simulink model "DescreteModel"  (R2020b)
settings: Solver=FixedStepAuto  StartTime=0.0  StopTime=5  FixedStep=0.0001  RelTol=1e-3
InitFcn:
  | run("NonLinearModelParameters")
  | 
  | run('model_disc_controller_creator.m')
values from neighbouring files (symbols this model uses):
  B = 3.4    [NonLinearModelParameters.m]
  K_tau = 42e-3    (= 0.042)    [NonLinearModelParameters.m]
  n_1 = 1/3    (= 0.333333333333)    [NonLinearModelParameters.m]
  r_3 = 0.01571    [NonLinearModelParameters.m]
undefined symbols (not defined in the file or in its folder): cont_den, cont_num, CoulombAndViscousFriction, CurrentOffset, Delta, discrete_constants, J_eq, SignOfVelocity, T_sample
libraries: simulink x1
settings Model: Creator=jonas  LastModifiedBy=Bens PC

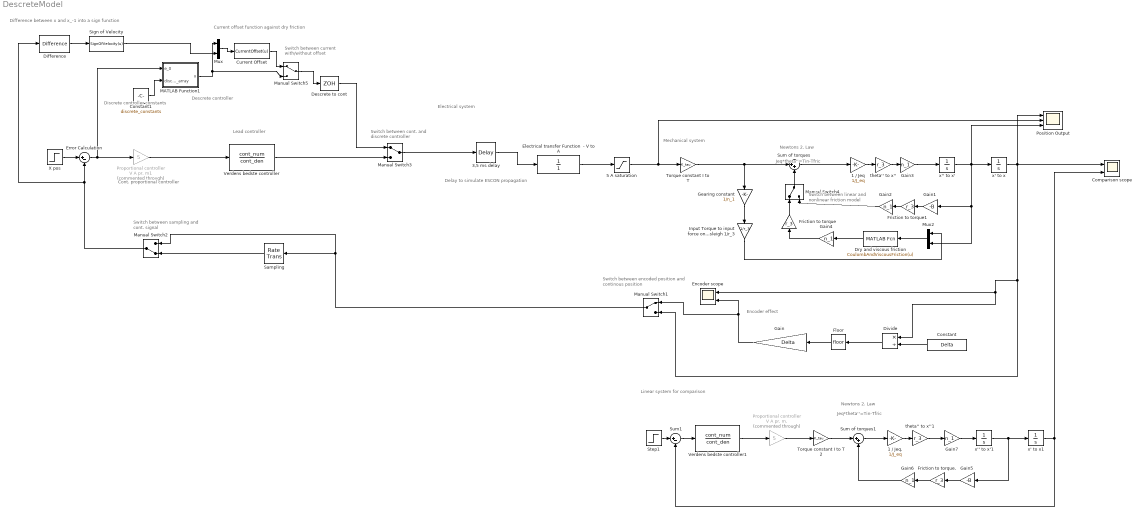
== system DescreteModel ==
  note: Discrete controller constants
  note: Difference between x and x_-1 into a sign function
  note: Linear system for comparison
  note: Switch between linear
      | and nonlinear friction model
  note: Delay to simulate ESCON propagation
  note: Switch between
      | current with/without offset
  note: Switch between sampling
      | and cont. signal
  note: Electrical system
  note: Switch between cont.
      | and discrete controller
  note: Current offset function against dry friction
  note: Cont. proportional
      | controller
  note: Switch between encoded position and
      | continous position
  note: Newtons 2. Law
  note: Mechanical system
  note: Encoder effect
  note: Jeq*theta''=Tin-Tfric
  note: Descrete controller
  note: Newtons 2. Law
  note: Jeq*theta''=Tin-Tfric
  note: Lead
      | controller
  1 / Jeq : Gain  Gain=1/J_eq
  1 / Jeq. : Gain  Gain=1/J_eq
  3,5 ms delay : TransportDelay  DelayTime=0.0035
  5 A saturation : Saturate  UpperLimit=5  LowerLimit=-5
  Comparison scope : Scope  NumInputPorts=2
  Constant : Constant  Value=Delta
  Constant1 : Constant  Value=discrete_constants
  Current Offset : MATLABFcn  MATLABFcn=CurrentOffset(u)  OutputDimensions=1
  Descrete to cont : ZeroOrderHold  SampleTime=T_sample
  Difference : simulink/Discrete/Difference  ICPrevInput=0.0  OutMin=[]  OutMax=[]  OutDataType=fixdt(1, 16)  OutScaling=2^-10  DoSatur=off
  Divide : Product  Inputs=*/
  Dry and viscous friction : MATLABFcn  MATLABFcn=CoulombAndViscousFriction(u)  OutputDimensions=1
  Electrical transfer Function  - V to A : TransferFcn  Denominator=[1]
  Encoder scope : Scope  NumInputPorts=2
  Error Calculation : Sum  Inputs=|+-
  Floor : Rounding
  Friction to torque : Gain  Gain=r_3
  Friction to torque. : Gain  Gain=r_3
  Friction to torque1 : Gain  Gain=r_3
  Gain : Gain  Gain=Delta
  Gain1 : Gain  Gain=-B
  Gain{2..4,6..7} (5 alike) : Gain  Gain=n_1
  Gain5 : Gain  Gain=-B
  Gearing constant : Gain  Gain=1/n_1
  Input Torque to input force on sleigh 1/r_3 : Gain  Gain=1/r_3
  MATLAB Function1 : MATLAB Function  TreatAsAtomicUnit=on
  Manual Switch{1,3..5} (4 alike) : ManualSwitch
  Manual Switch2 : ManualSwitch  CurrentSetting=0
  Mux : Mux  Inputs=2
  Mux2 : Mux  Inputs=2
  Position Output : Scope  NumInputPorts=3
  Proportional controller V A pr. m. : Gain  Commented=through  Gain=5
  Proportional controller V A pr. m1 : Gain  Commented=through  Gain=5
  "Sampling " : RateTransition  OutPortSampleTime=T_sample
  Sign of Velocity : MATLABFcn  MATLABFcn=SignOfVelocity(u)  OutputDimensions=1
  Step1 : Step  Time=0  After=0.5  SampleTime=0
  Sum of torques : Sum  Inputs=|++
  Sum of torques1 : Sum  Inputs=|++
  Sum1 : Sum  Inputs=|+-
  "Torque constant I to T " : Gain  Gain=K_tau
  Torque constant I to T 2 : Gain  Gain=K_tau
  Verdens bedste controller : TransferFcn  Numerator=cont_num  Denominator=cont_den
  Verdens bedste controller1 : TransferFcn  Numerator=cont_num  Denominator=cont_den
  X pos : Step  Time=0  After=0.5  SampleTime=0
  theta'' to x'' : Gain  Gain=r_3
  theta'' to x''1 : Gain  Gain=r_3
  x' to x : Integrator
  x' to x1 : Integrator
  x'' to x' : Integrator
  x'' to x'1 : Integrator
  wires:
  Sum of torques/1 -> 1 / Jeq/1
  theta'' to x''/1 -> Gain3/1
  X pos/1 -> Error Calculation/1
  x'' to x'/1 -> Position Output/3, Gain1/1, Mux2/2, x' to x/1
  Electrical transfer Function  - V to A/1 -> 5 A saturation/1
  Input Torque to input force on sleigh 1/r_3/1 -> Mux2/1
  Mux2/1 -> Dry and viscous friction/1
  5 A saturation/1 -> Position Output/2, "Torque constant I to T "/1
  Gain/1 -> Encoder scope/2, Manual Switch1/1
  Floor/1 -> Gain/1
  Constant/1 -> Divide/2
  Manual Switch3/1 -> 3,5 ms delay/1
  Divide/1 -> Floor/1
  Manual Switch1/1 -> "Sampling "/1, Manual Switch2/1
  "Sampling "/1 -> Manual Switch2/2
  Descrete to cont/1 -> Manual Switch3/1
  Proportional controller V A pr. m1/1 -> Verdens bedste controller/1
  Dry and viscous friction/1 -> Gain4/1
  3,5 ms delay/1 -> Electrical transfer Function  - V to A/1
  1 / Jeq/1 -> theta'' to x''/1
  Manual Switch4/1 -> Sum of torques/2
  Friction to torque/1 -> Manual Switch4/1
  Gain1/1 -> Friction to torque1/1
  Friction to torque1/1 -> Gain2/1
  "Torque constant I to T "/1 -> Sum of torques/1, Gearing constant/1
  Gearing constant/1 -> Input Torque to input force on sleigh 1/r_3/1
  Gain2/1 -> Manual Switch4/2
  Gain3/1 -> x'' to x'/1
  Gain4/1 -> Friction to torque/1
  Friction to torque./1 -> Gain6/1
  Gain7/1 -> x'' to x'1/1
  Gain5/1 -> Friction to torque./1
  x'' to x'1/1 -> Gain5/1, x' to x1/1
  Gain6/1 -> Sum of torques1/2
  1 / Jeq./1 -> theta'' to x''1/1
  Sum of torques1/1 -> 1 / Jeq./1
  Sum1/1 -> Verdens bedste controller1/1
  Step1/1 -> Sum1/1
  Torque constant I to T 2/1 -> Sum of torques1/1
  x' to x/1 -> Comparison scope/1, Divide/1, Encoder scope/1, Manual Switch1/2, Position Output/1
  x' to x1/1 -> Comparison scope/2, Sum1/2
  Proportional controller V A pr. m./1 -> Torque constant I to T 2/1
  Verdens bedste controller1/1 -> Proportional controller V A pr. m./1
  theta'' to x''1/1 -> Gain7/1
  Manual Switch5/1 -> Descrete to cont/1
  Current Offset/1 -> Manual Switch5/1
  Mux/1 -> Current Offset/1
  Sign of Velocity/1 -> Mux/2
  Manual Switch2/1 -> Difference/1, Error Calculation/2
  Difference/1 -> Sign of Velocity/1
  MATLAB Function1/1(u) -> Mux/1, Manual Switch5/2
  Verdens bedste controller/1 -> Manual Switch3/2
  Error Calculation/1 -> Proportional controller V A pr. m1/1, MATLAB Function1/1(e_0)
  Constant1/1 -> MATLAB Function1/2(discrete_array)

== matlab function DescreteModel/MATLAB Function1 ==
  settings: updateMethod=DISCRETE  sampleTime=T_sample
  data: e_0 input; u output; discrete_array input
function u = Controller(e_0, discrete_array)
persistent u_1 e_1 e_2 e_3 e_4 u_2 u_3 u_4 ;

coder.extrinsic('evalin', 'assignin') %% this allows access to T_sample
T = 0;
T = evalin('base','T_sample'); % Read value from workspace



%% discrete array input has the following format
%discrete_array(1) =  u_n FD array 
%discrete_array(2) =  e_n FD array 
%discrete_array(3) =  u_n BD array 
%discrete_array(4) =  e_n BD array 




%% With a FD controller
u_n_array = discrete_array(3, 1:end);
e_n_array = discrete_array(4, 1:end);











% Continuous controller : 
%tf_numerator = [1.203 3.6];
%tf_denomenator = [0.04812 1];




%Discrete output from program














if isempty(e_1)
    e_1 = 0;
end
if isempty(e_2)
    e_2 = 0;
end
if isempty(e_3)
    e_3 = 0;
end
if isempty(u_1)
    u_1 = 0;
end

if isempty(u_2)
    u_2 = 0;
end
if isempty(u_3)
    u_3 = 0;
end
if isempty(e_4)
    e_4 = 0;
end
if isempty(u_4)
    u_4 = 0;
end





e_n_length = length(e_n_array);
u_n_length = length(u_n_array); 

if e_n_length == 1
    e_n_equation = e_0 * e_n_array(1);
elseif e_n_length ==2
        e_n_equation = e_0 * e_n_array(1) + e_1 * e_n_array(2);
elseif e_n_length ==3
        e_n_equation = e_0 * e_n_array(1) + e_n_array(2) * e_1 + e_2 * e_n_array(3);
elseif e_n_length ==4
        e_n_equation = e_0 * e_n_array(1) + e_n_array(2) * e_1 + e_2 * e_n_array(3) + e_3 * e_n_array(4);
else
    e_n_equation = 0
end

if u_n_length == 1
        u_n_equation = u_1 * u_n_array(1);
elseif u_n_length == 2
        u_n_equation = u_1 * u_n_array(1) + u_2 * u_n_array(2);
elseif u_n_length ==3
        u_n_equation = u_1 * u_n_array(1) + u_n_array(2) * u_2 + u_3 * u_n_array(3);
elseif u_n_length ==4
        u_n_equation = u_1 * u_n_array(1) + u_n_array(2) * u_2 + u_3 * u_n_array(3) + u_4 * u_n_array(4);
else
    u_n_equation = 0;
end



u = e_n_equation + u_n_equation;

%u = (1447209*e_2 + 1203000*T*u_1 - e_1*(30075000*T + 2894418) + e_0*(90000000*T^2 + 30075000*T + 1447209))/(1000*T*(25000*T + 1203));

e_3 = e_2;
e_2=e_1;
e_1=e_0;

u_4 = u_3;
u_3 = u_2;
u_2 = u_1;

u_1=u;

end
